simulink model "ATABEY_sistem_modeli"  (R2025b)
settings: Solver=VariableStepAuto  StartTime=0.0  StopTime=simTime  RelTol=1e-3
undefined symbols (not defined in the file): u1max, u1min, u2max, u2min, u3max, u3min, u4max, u4min, x0
libraries: sharedTrackingLibrary x1, aerolibfltsims x1, aerolibanimutils x1
settings Model: Creator=erayacikgz  LastModifiedBy=erayacikgz

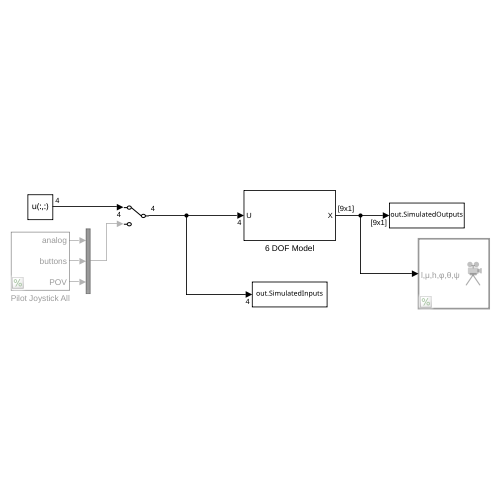
[thumbnail: Simulink's stored preview of the top-level diagram]
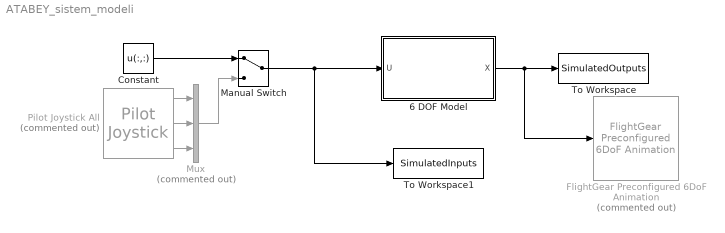
== system ATABEY_sistem_modeli ==
  6 DOF Model : Subsystem
  Constant : Constant  Value=u(:,:)
  FlightGear Preconfigured 6DoF Animation : aerolibfltsims/FlightGear Preconfigured 6DoF Animation  Commented=on  xFlightGearVersion=v2019.1  DestinationIpAddress=127.0.0.1  DestinationPort=5502  SampleTime=1/30  packetVersion=24
  Manual Switch : ManualSwitch
  Mux : Mux  Commented=on  Inputs=3
  Pilot Joystick All : aerolibanimutils/Pilot Joystick  Commented=on  JoystickID=Joystick1  OutputConfiguration=AllOutputs  SampleTime=1/30
      settings: LibrarySourceBlock=aerolibanimutils/Pilot Joystick All
  To Workspace : ToWorkspace  VariableName=SimulatedOutputs  SaveFormat=Timeseries  SampleTime=-1
  To Workspace1 : ToWorkspace  VariableName=SimulatedInputs  SaveFormat=Timeseries  SampleTime=-1
  wires:
  6 DOF Model/1(X) -> FlightGear Preconfigured 6DoF Animation/1, To Workspace/1
  Manual Switch/1 -> To Workspace1/1, 6 DOF Model/1(U)
  Constant/1 -> Manual Switch/1
  Pilot Joystick All/1 -> Mux/1
  Pilot Joystick All/2 -> Mux/2
  Pilot Joystick All/3 -> Mux/3
  Mux/1 -> Manual Switch/2

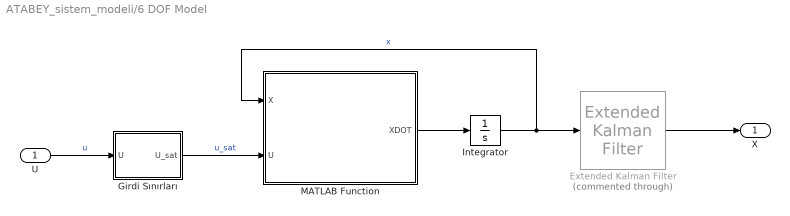
== system ATABEY_sistem_modeli/6 DOF Model ==
  U : Inport
  Extended Kalman Filter : sharedTrackingLibrary/Extended Kalman Filter  Commented=through  StateTransitionFcn=myStateTransitionFcn  HasStateTransitionJacobianFcn=off  HasAdditiveProcessNoise=Additive  ProcessNoise=1  HasTimeVaryingProcessNoise=off  HasStateTransitionFcnExtraArgument=0  InitialState=0  InitialStateCovariance=1  MeasurementFcn1=myMeasurementFcn  HasMeasurementJacobianFcn1=off  HasMeasurementEnablePort1=off  HasAdditiveMeasurementNoise1=Additive  MeasurementNoise1=1  HasTimeVaryingMeasurementNoise1=off  HasMeasurementFcnExtraArgument1=0  HasMeasurementWrapping1=off  MeasurementFcn2=myMeasurementFcn  HasMeasurementJacobianFcn2=off  HasMeasurementEnablePort2=off  HasAdditiveMeasurementNoise2=Additive  MeasurementNoise2=1  HasTimeVaryingMeasurementNoise2=off  HasMeasurementFcnExtraArgument2=0  HasMeasurementWrapping2=off  MeasurementFcn3=myMeasurementFcn  HasMeasurementJacobianFcn3=off  HasMeasurementEnablePort3=off  HasAdditiveMeasurementNoise3=Additive  MeasurementNoise3=1  HasTimeVaryingMeasurementNoise3=off  HasMeasurementFcnExtraArgument3=0  HasMeasurementWrapping3=off  MeasurementFcn4=myMeasurementFcn  HasMeasurementJacobianFcn4=off  HasMeasurementEnablePort4=off  HasAdditiveMeasurementNoise4=Additive  MeasurementNoise4=1  HasTimeVaryingMeasurementNoise4=off  HasMeasurementFcnExtraArgument4=0  HasMeasurementWrapping4=off  MeasurementFcn5=myMeasurementFcn  HasMeasurementJacobianFcn5=off  HasMeasurementEnablePort5=off  HasAdditiveMeasurementNoise5=Additive  MeasurementNoise5=1  HasTimeVaryingMeasurementNoise5=off  HasMeasurementFcnExtraArgument5=0  HasMeasurementWrapping5=off  EnableMultirate=off  StateTransitionFcnSampleTime=1  MeasurementFcn1SampleTime=1  MeasurementFcn2SampleTime=1  MeasurementFcn3SampleTime=1  MeasurementFcn4SampleTime=1  MeasurementFcn5SampleTime=1  UseCurrentEstimator=on  OutputStateCovariance=off  DataType=double  SampleTime=1  NumberOfMeasurements=1
  Girdi Sınırları : Subsystem
  Integrator : Integrator  InitialCondition=x0(:,:)
  MATLAB Function : MATLAB Function  TreatAsAtomicUnit=on
  X : Outport
  wires:
  MATLAB Function/1(XDOT) -> Integrator/1
  U/1 -> Girdi Sınırları/1(U)  "u"
  Girdi Sınırları/1(U_sat) -> MATLAB Function/2(U)  "u_sat"
  Integrator/1 -> MATLAB Function/1(X), Extended Kalman Filter/1  "x"
  Extended Kalman Filter/1 -> X/1

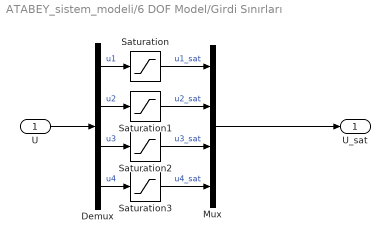
== system ATABEY_sistem_modeli/6 DOF Model/Girdi Sınırları ==
  U : Inport
  Demux : Demux
  Mux : Mux
  Saturation : Saturate  UpperLimit=u1max  LowerLimit=u1min
  Saturation1 : Saturate  UpperLimit=u2max  LowerLimit=u2min
  Saturation2 : Saturate  UpperLimit=u3max  LowerLimit=u3min
  Saturation3 : Saturate  UpperLimit=u4max  LowerLimit=u4min
  U_sat : Outport
  wires:
  Saturation2/1 -> Mux/3  "u3_sat"
  Mux/1 -> U_sat/1
  Demux/2 -> Saturation1/1  "u2"
  Demux/4 -> Saturation3/1  "u4"
  Saturation1/1 -> Mux/2  "u2_sat"
  Saturation/1 -> Mux/1  "u1_sat"
  Saturation3/1 -> Mux/4  "u4_sat"
  Demux/3 -> Saturation2/1  "u3"
  U/1 -> Demux/1
  Demux/1 -> Saturation/1  "u1"

== matlab function ATABEY_sistem_modeli/6 DOF Model/MATLAB Function ==
  data: X input double size=[9 1]; XDOT output double size=[9 1]; U input double size=[4 1]
function XDOT = ATABEY_model(X, U)

    XDOT = ATABEY_dynamics(X, U);
    
end
